simulink model "CE_SEE_Final"  (R2025a)
settings: Solver=VariableStepAuto  StartTime=0.0  StopTime=0.2  RelTol=1e-3
libraries: dspsrcs4 x4, commchan3 x3, dspfdesign x3
settings Model: Creator=Shreya  LastModifiedBy=Sidharth Ghosh

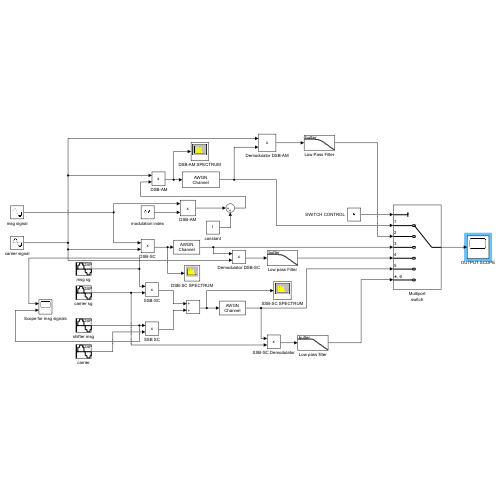
[thumbnail: Simulink's stored preview of the top-level diagram]
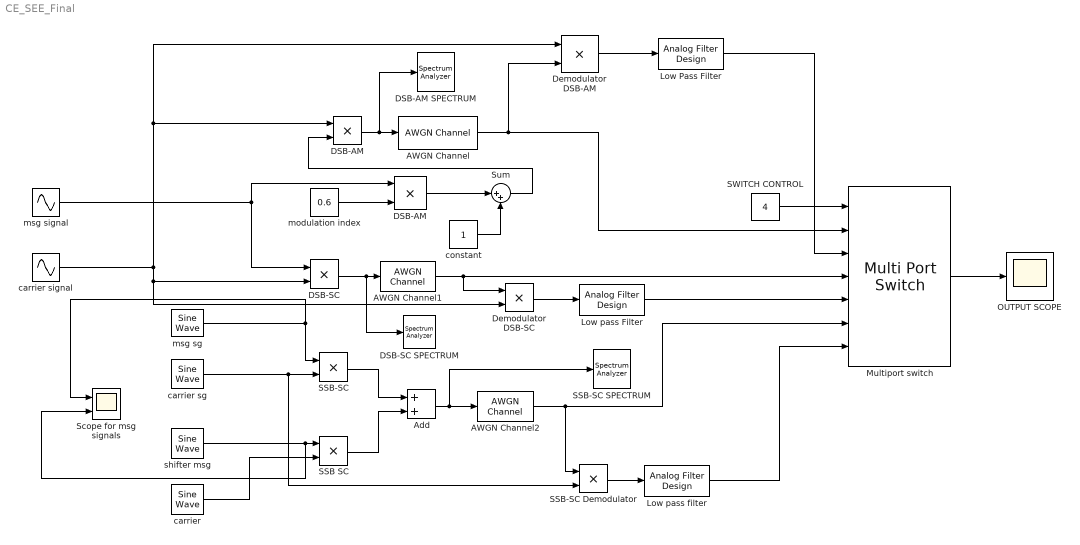
== system CE_SEE_Final ==
  " DSB-AM" : Product
  AWGN Channel : commchan3/AWGN Channel  LegacyMode=off  NoiseMethod="Signal to noise ratio  (SNR)"  noiseMode="Signal to noise ratio  (SNR)"  EbNo=10  EsNo=10  SNR=30  BitsPerSymbol=1  SignalPower=1  SpecifySymbolPeriod=off  SamplesPerSymbol=1  SymbolPeriod=1  VarianceSource=Parameter  Variance=1  RandomStream=Global stream  Seed=67  SimulateUsing=Code generation
  AWGN Channel1 : commchan3/AWGN Channel  LegacyMode=off  NoiseMethod="Signal to noise ratio  (SNR)"  noiseMode="Signal to noise ratio  (SNR)"  EbNo=10  EsNo=10  SNR=30  BitsPerSymbol=1  SignalPower=1  SpecifySymbolPeriod=off  SamplesPerSymbol=1  SymbolPeriod=1  VarianceSource=Parameter  Variance=1  RandomStream=Global stream  Seed=67  SimulateUsing=Code generation
  AWGN Channel2 : commchan3/AWGN Channel  LegacyMode=off  NoiseMethod="Signal to noise ratio  (SNR)"  noiseMode="Signal to noise ratio  (SNR)"  EbNo=10  EsNo=10  SNR=20  BitsPerSymbol=1  SignalPower=1  SpecifySymbolPeriod=off  SamplesPerSymbol=1  SymbolPeriod=1  VarianceSource=Parameter  Variance=1  RandomStream=Global stream  Seed=67  SimulateUsing=Code generation
  Add : Sum
  DSB-AM : Product
  DSB-AM SPECTRUM : SpectrumAnalyzer  WindowPosition=[1.000000,379.000000,400.000000,334.000000,]  Visible=on  ScopeFrameLocation=window  WindowInvariantSamplesPerUpdate=on  Span=20000  StartFrequency=-10000  StopFrequency=10000  YLimits=[-37.1509 36.9052]
  DSB-SC : Product
  DSB-SC SPECTRUM : SpectrumAnalyzer  WindowPosition=[760.000000,377.000000,401.000000,327.000000,]  Visible=on  ScopeFrameLocation=window  WindowInvariantSamplesPerUpdate=on  Span=20000  StartFrequency=-10000  StopFrequency=10000  YLimits=[-41.6944 31.2538]
  Demodulator DSB-AM : Product
  Demodulator DSB-SC : Product
  Low Pass Filter : dspfdesign/Analog Filter Design  method=Butterworth  filttype=Lowpass  N=2  Wlo=942.5  Whi=80  Rp=2  Rs=40
  Low pass Filter : dspfdesign/Analog Filter Design  method=Butterworth  filttype=Lowpass  N=2  Wlo=942.5  Whi=80  Rp=2  Rs=40
  Low pass filter : dspfdesign/Analog Filter Design  method=Butterworth  filttype=Lowpass  N=20  Wlo=2*pi*1000  Whi=80  Rp=2  Rs=40
  Multiport switch : MultiPortSwitch  Inputs=6  SaturateOnIntegerOverflow=off  InputSameDT=off
  OUTPUT SCOPE : Scope
      settings: ActiveDisplayYMinimum=-25.410724888662145  ActiveDisplayYMaximum=25.286708532080453
  SSB SC : Product
  SSB-SC : Product
  SSB-SC Demodulator : Product
  SSB-SC SPECTRUM : SpectrumAnalyzer  WindowPosition=[-1.000000,28.000000,408.000000,321.000000,]  Visible=on  ScopeFrameLocation=window  WindowInvariantSamplesPerUpdate=on  Span=20000  StartFrequency=-10000  StopFrequency=10000  YLimits=[-35.031 56.2696]
  SWITCH CONTROL : Constant  Value=4
  Scope for msg signals : Scope  NumInputPorts=2
      settings: ActiveDisplayYMinimum=-5.3272360362890723  ActiveDisplayYMaximum=5.5077876292345787  DataLoggingVariableName=ScopeData4
  Sum : Sum  Inputs=|++
  carrier : dspsrcs4/Sine Wave  Amplitude=3  Frequency=1000  Phase=pi/2  SampleMode=Discrete  OutComplex=Real  CompMethod=Trigonometric fcn  TableSize=Speed  SampleTime=1/10000  SamplesPerFrame=1  ResetState=Restart at time zero  OutputFrames=off  dataType=double  wordLen=16  udDataType=sfix(16)  fracBitsMode=Best precision  numFracBits=15  OutDataTypeStr=double  LastOutDataTypeStr=double
  carrier sg : dspsrcs4/Sine Wave  Amplitude=3  Frequency=1000  Phase=0  SampleMode=Discrete  OutComplex=Real  CompMethod=Trigonometric fcn  TableSize=Speed  SampleTime=1/10000  SamplesPerFrame=1  ResetState=Restart at time zero  OutputFrames=off  dataType=double  wordLen=16  udDataType=sfix(16)  fracBitsMode=Best precision  numFracBits=15  OutDataTypeStr=double  LastOutDataTypeStr=double
  carrier signal : Sin  Amplitude=2  Frequency=2*pi*1000  Phase=pi/2  SampleTime=1/20000
  constant : Constant
  modulation index : Constant  Value=0.6
  msg sg : dspsrcs4/Sine Wave  Amplitude=5  Frequency=100  Phase=0  SampleMode=Discrete  OutComplex=Real  CompMethod=Trigonometric fcn  TableSize=Speed  SampleTime=1/10000  SamplesPerFrame=1  ResetState=Restart at time zero  OutputFrames=off  dataType=double  wordLen=16  udDataType=sfix(16)  fracBitsMode=Best precision  numFracBits=15  OutDataTypeStr=double  LastOutDataTypeStr=double
  msg signal : Sin  Frequency=2*pi*100  Samples=100  SampleTime=1/20000
  shifter msg : dspsrcs4/Sine Wave  Amplitude=5  Frequency=100  Phase=pi/2  SampleMode=Discrete  OutComplex=Real  CompMethod=Trigonometric fcn  TableSize=Speed  SampleTime=1/10000  SamplesPerFrame=1  ResetState=Restart at time zero  OutputFrames=off  dataType=double  wordLen=16  udDataType=sfix(16)  fracBitsMode=Best precision  numFracBits=15  OutDataTypeStr=double  LastOutDataTypeStr=double
  wires:
  msg signal/1 -> DSB-AM/1, DSB-SC/1
  carrier signal/1 -> Demodulator DSB-AM/1, " DSB-AM"/1, Demodulator DSB-SC/2, DSB-SC/2
  constant/1 -> Sum/2
  DSB-AM/1 -> Sum/1
  modulation index/1 -> DSB-AM/2
  SWITCH CONTROL/1 -> Multiport switch/1
  Sum/1 -> " DSB-AM"/2
  " DSB-AM"/1 -> DSB-AM SPECTRUM/1, AWGN Channel/1
  DSB-SC/1 -> DSB-SC SPECTRUM/1, AWGN Channel1/1
  Demodulator DSB-SC/1 -> Low pass Filter/1
  Low pass Filter/1 -> Multiport switch/5
  Low Pass Filter/1 -> Multiport switch/3
  Multiport switch/1 -> OUTPUT SCOPE/1
  Demodulator DSB-AM/1 -> Low Pass Filter/1
  AWGN Channel1/1 -> Multiport switch/4, Demodulator DSB-SC/1
  AWGN Channel/1 -> Multiport switch/2, Demodulator DSB-AM/2
  SSB-SC/1 -> Add/1
  SSB SC/1 -> Add/2
  carrier sg/1 -> SSB-SC/2, SSB-SC Demodulator/2
  shifter msg/1 -> Scope for msg signals/2, SSB SC/1
  carrier/1 -> SSB SC/2
  Add/1 -> AWGN Channel2/1, SSB-SC SPECTRUM/1
  SSB-SC Demodulator/1 -> Low pass filter/1
  Low pass filter/1 -> Multiport switch/7
  AWGN Channel2/1 -> SSB-SC Demodulator/1, Multiport switch/6
  msg sg/1 -> SSB-SC/1, Scope for msg signals/1
